simulink model "FULL_IM_HESS"  (R2017b)
settings: Solver=ode4  StartTime=0.0  StopTime=SIMULPARAM.T_end  FixedStep=SIMULPARAM.Ts  RelTol=1e-3  EnableMultiTasking=on
undefined symbols (not defined in the file): BAT, Bat_current_control, BATCURRENTCONTROL, CHAS, Chopper, d_current_control, DC_bus_voltage_control, DCBUSCONTROL, DCCAP, dCURRENTCONTROL, ENV, Flux_control, FLUXCONTROL, FLUXSTRATEGY, IM, L, q_current_control, qCURRENTCONTROL, SC, SC_current_control, SCCURRENTCONTROL, Speed_control, SPEEDCONTROL, STRATEGY, TRANS
libraries: simulink x3
(part 1 of 2)
settings Model: Creator=Huy  LastModifiedBy=baohu
settings DataIOCC: SaveFormat=Array  SignalLoggingSaveFormat=ModelDataLogs  SaveOutput=off  SignalLogging=off  SaveTime=off
settings OptimizationCC: ExpressionDepthLimit=2147483647  LifeSpan=inf
settings DebuggingCC: AlgebraicLoopMsg=none  SaveWithDisabledLinksMsg=none  UnderspecifiedInitializationDetection=Classic  MergeDetectMultiDrivingBlocksExec=none  MaxConsecutiveZCsMsg=none  SolverPrmCheckMsg=warning  FcnCallInpInsideContextMsg=warning  ModelReferenceDataLoggingMessage=none  ModelReferenceExtraNoncontSigs=none  StateNameClashWarn=warning  SFUnexpectedBacktrackingDiag=warning  SFNoUnconditionalDefaultTransitionDiag=warning  SFExecutionAtInitializationDiag=none
settings HardwareCC: ProdBitPerPointer=32  ProdBitPerSizeT=32  ProdBitPerPtrDiffT=32  ProdLargestAtomicFloat=None  ProdIntDivRoundTo=Undefined  ProdEndianess=Unspecified  ProdWordSize=32  ProdHWDeviceType=32-bit Generic
settings ModelReferenceCC: PropagateSignalLabelsOutOfModel=off
settings CodeAppCC: StateflowObjectComments=on
settings GRTTargetCC: TargetLangStandard=C89/C90 (ANSI)  CombineOutputUpdateFcns=off  GRTInterface=on
settings ConfigComp: CovMetricSettings=dw  CovHtmlReporting=on  CovSaveCumulativeToWorkspaceVar=on  CovSaveSingleToWorkspaceVar=on  CovExternalEMLEnable=off

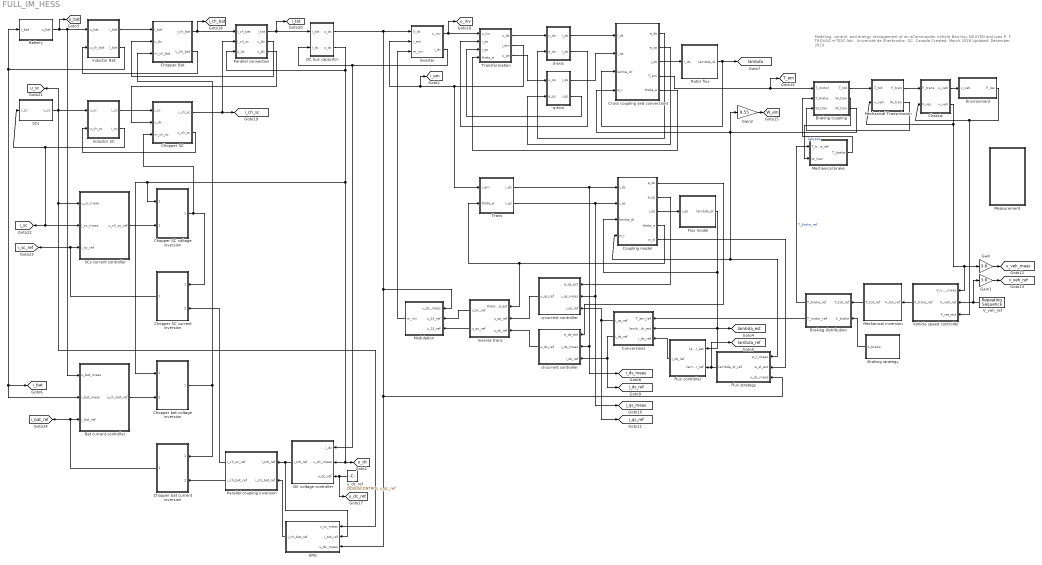
== system FULL_IM_HESS ==
  note: Modeling, control, and energy management of an eCommander vehicle
      | Bao-Huy NGUYEN and Joao P. F. TROVAO
      | e-TESC lab., Université de Sherbrooke, QC, Canada
      | Created: March 2018 Updated: December 2019
  Bat current controller : Subsystem
      mask Display: plot(0,0,100,100, [10,30,90,70,10,90],[90,10,10,90,90,10])
  Battery : Subsystem  AncestorBlock=simulink/REM/SE
      mask Display:
      | plot(0,0,100,100, 1.2*[50,57.68,60.77,63.08,64.97,66.58,68,69.26,70.4, 	71.42,72.36,78.28,80,78.28,72.36,71.42,70.4, 	69.26,68,66.58,64.97,63.08,60.77,57.68,50,42.32, 	39.23,36.92,35.03,33.42,32,30.74,29.6,28.58, 	27.64,21.72,20,21.72,27.64,28.58,29.6,30.74,32, 	33.42,35.03,36.92,39.23,42.32,50]-10, 1.2*[20,21,22,23,24,25,26,27,28,29,30,40,50,60,70,71,72, 	73,74,75,76,77,78,79,80,79,78,77,76,75,74,73,72, 	71,70,60,50,40,30,29,28,27,26,25,24,23,22,21,20]-10)
      | disp('ES')
  Braking coupling : Subsystem  mask(CM){}
      mask Display: plot(0,0,100,100,[35,35,95,95,35],[65,10,10,65,65], [5,5,65,65,5],[90,35,35,90,90])
  Braking distribution : Subsystem  AncestorBlock=simulink/SMC/Bloc de répartition
      mask Display: plot(0,0,100,100,[20,40,100,80,20],[75,20,20,75,75], [0,20,80,60,0],[85,30,30,85,85])
  Braking strategy : Subsystem  AncestorBlock=simulink/SMC/Inversion EC avec mesure
      mask Display: plot(0,0,100,100,[10,30,90,70,10],[90,10,10,90,90])
  Chassis : Subsystem  AncestorBlock=simulink/REM/EA  mask(CM){}
      mask Display: plot(0,0,100,100,[10,10,90,90,10],[90,10,10,90,90], [10,90],[10,90])
  Chopper Bat : Subsystem  AncestorBlock=simulink/REM/EC Elec  mask(Hacheur){}
      mask Display: plot(0,0,100,100,[10,10,90,90,10],[90,10,10,90,90])
  Chopper SC : Subsystem  AncestorBlock=simulink/REM/EC Elec  mask(Hacheur){}
      mask Display: plot(0,0,100,100,[10,10,90,90,10],[90,10,10,90,90])
  Chopper SC current inversion : Subsystem
      mask Display: plot(0,0,100,100,[10,30,90,70,10],[90,10,10,90,90])
  Chopper SC voltage inversion : Subsystem
      mask Display: plot(0,0,100,100,[10,30,90,70,10],[90,10,10,90,90])
  Chopper bat current inversion : Subsystem
      mask Display: plot(0,0,100,100,[10,30,90,70,10],[90,10,10,90,90])
  Chopper bat voltage inversion : Subsystem
      mask Display: plot(0,0,100,100,[10,30,90,70,10],[90,10,10,90,90])
  Conversions : Subsystem  AncestorBlock=simulink/SMC/Bloc de répartition
      mask Display: plot(0,0,100,100,[20,40,100,80,20],[75,20,20,75,75], [0,20,80,60,0],[85,30,30,85,85])
  Coupling model : Subsystem  AncestorBlock=simulink/REM/EC EM
      mask Display: plot(0,0,100,100, [50,57.68,60.77,63.08,64.97,66.58,68,69.26,70.4, 	71.42,72.36,78.28,80,78.28,72.36,71.42,70.4, 	69.26,68,66.58,64.97,63.08,60.77,57.68,50,42.32, 	39.23,36.92,35.03,33.42,32,30.74,29.6,28.58, 	27.64,21.72,20,21.72,27.64,28.58,29.6,30.74,32, 	33.42,35.03,36.92,39.23,42.32,50], [20,21,22,23,24,25,26,27,28,29,30,40,50,60,70,71,72, 	73,74,75,76,77,78,79,80,79,78,77,76,75,74,73,72, 	71,70,60,50,40,30,29,28,27,26,25,24,23,22,21,20]-15,  [50,57.68,60.77,63.08,64.97,66.58,68,69.26,70.4, 	71.42,72.36,78.28,80,78.28,72.36,71.42,70.4, 	69.26,68,66.58,64.97,63.08,60.77,57.68,50,42.32, 	39.23,36.92,35.03,33.42,32,30.74,29.6,28.58, 	27.64,21.72,20,21.72,27.64,28.58,29.6,30.74,32, 	33.42,35.03,36.92,39.23,42.32,50], [20,21,22,23,24,25,26,27,28,29,30,40,50,60,70,71,72, 	73,74,75,76,77,78,79,80,79,78,77,76,75,74,73,72, 	71,70,60,50,40,30,29,28,27,26,25,24,23,22,21,20]+15)
  Cross coupling and conversions : Subsystem  mask(CM){}
      mask Display: plot(0,0,100,100, [50,57.68,60.77,63.08,64.97,66.58,68,69.26,70.4, 	71.42,72.36,78.28,80,78.28,72.36,71.42,70.4, 	69.26,68,66.58,64.97,63.08,60.77,57.68,50,42.32, 	39.23,36.92,35.03,33.42,32,30.74,29.6,28.58, 	27.64,21.72,20,21.72,27.64,28.58,29.6,30.74,32, 	33.42,35.03,36.92,39.23,42.32,50], [20,21,22,23,24,25,26,27,28,29,30,40,50,60,70,71,72, 	73,74,75,76,77,78,79,80,79,78,77,76,75,74,73,72, 	71,70,60,50,40,30,29,28,27,26,25,24,23,22,21,20]-15,  [50,57.68,60.77,63.08,64.97,66.58,68,69.26,70.4, 	71.42,72.36,78.28,80,78.28,72.36,71.42,70.4, 	69.26,68,66.58,64.97,63.08,60.77,57.68,50,42.32, 	39.23,36.92,35.03,33.42,32,30.74,29.6,28.58, 	27.64,21.72,20,21.72,27.64,28.58,29.6,30.74,32, 	33.42,35.03,36.92,39.23,42.32,50], [20,21,22,23,24,25,26,27,28,29,30,40,50,60,70,71,72, 	73,74,75,76,77,78,79,80,79,78,77,76,75,74,73,72, 	71,70,60,50,40,30,29,28,27,26,25,24,23,22,21,20]+15)
  DC bus capacitor : Subsystem  AncestorBlock=simulink/REM/EA  mask(CM){}
      mask Display: plot(0,0,100,100,[10,10,90,90,10],[90,10,10,90,90], [10,90],[10,90])
  DC voltage controller : Subsystem  AncestorBlock=simulink/SMC/Asservissement Correcteur IP
      mask Display: plot(0,0,100,100, [10,30,90,70,10,90],[90,10,10,90,90,10])
  EMS : Subsystem  AncestorBlock=simulink/SMC/Inversion EC avec mesure
      mask Display: plot(0,0,100,100,[10,30,90,70,10],[90,10,10,90,90])
  Environment : Subsystem  AncestorBlock=simulink/REM/SE
      mask Display:
      | plot(0,0,100,100, 1.2*[50,57.68,60.77,63.08,64.97,66.58,68,69.26,70.4, 	71.42,72.36,78.28,80,78.28,72.36,71.42,70.4, 	69.26,68,66.58,64.97,63.08,60.77,57.68,50,42.32, 	39.23,36.92,35.03,33.42,32,30.74,29.6,28.58, 	27.64,21.72,20,21.72,27.64,28.58,29.6,30.74,32, 	33.42,35.03,36.92,39.23,42.32,50]-10, 1.2*[20,21,22,23,24,25,26,27,28,29,30,40,50,60,70,71,72, 	73,74,75,76,77,78,79,80,79,78,77,76,75,74,73,72, 	71,70,60,50,40,30,29,28,27,26,25,24,23,22,21,20]-10)
      | disp('MS')
  Flux controller : Subsystem  AncestorBlock=simulink/SMC/Asservissement Correcteur IP
      mask Display: plot(0,0,100,100, [10,30,90,70,10,90],[90,10,10,90,90,10])
  Flux model : Subsystem  AncestorBlock=simulink/REM/EA  mask(CM){}
      mask Display: plot(0,0,100,100,[10,10,90,90,10],[90,10,10,90,90], [10,90],[10,90])
  Flux strategy : Subsystem  AncestorBlock=simulink/SMC/Inversion EC avec mesure
      mask Display: plot(0,0,100,100,[10,30,90,70,10],[90,10,10,90,90])
  Gain : Gain  Gain=3.6
  Gain1 : Gain  Gain=3.6
  Gain2 : Gain  Gain=9.55
  Inductor Bat : Subsystem  AncestorBlock=simulink/REM/EA  mask(CM){}
      mask Display: plot(0,0,100,100,[10,10,90,90,10],[90,10,10,90,90], [10,90],[10,90])
  Inductor SC : Subsystem  AncestorBlock=simulink/REM/EA  mask(CM){}
      mask Display: plot(0,0,100,100,[10,10,90,90,10],[90,10,10,90,90], [10,90],[10,90])
  Inverse trans : Subsystem  AncestorBlock=simulink/SMC/Bloc de répartition
      mask Display: plot(0,0,100,100,[20,40,100,80,20],[75,20,20,75,75], [0,20,80,60,0],[85,30,30,85,85])
  Inverter : Subsystem  AncestorBlock=simulink/REM/EC Elec  mask(Hacheur){}
      mask Display: plot(0,0,100,100,[10,10,90,90,10],[90,10,10,90,90])
  Measurement : Subsystem
  Mechanical Transmission : Subsystem
      mask Display: plot(0,0,100,100,[10,10,90,90,10],[90,10,10,90,90])
  Mechanical brake : Subsystem  AncestorBlock=simulink/REM/SE
      mask Display:
      | plot(0,0,100,100, 1.2*[50,57.68,60.77,63.08,64.97,66.58,68,69.26,70.4, 	71.42,72.36,78.28,80,78.28,72.36,71.42,70.4, 	69.26,68,66.58,64.97,63.08,60.77,57.68,50,42.32, 	39.23,36.92,35.03,33.42,32,30.74,29.6,28.58, 	27.64,21.72,20,21.72,27.64,28.58,29.6,30.74,32, 	33.42,35.03,36.92,39.23,42.32,50]-10, 1.2*[20,21,22,23,24,25,26,27,28,29,30,40,50,60,70,71,72, 	73,74,75,76,77,78,79,80,79,78,77,76,75,74,73,72, 	71,70,60,50,40,30,29,28,27,26,25,24,23,22,21,20]-10)
      | disp('MS')
  Mechanical inversion : Subsystem  AncestorBlock=simulink/SMC/Inversion EC avec mesure
      mask Display: plot(0,0,100,100,[10,30,90,70,10],[90,10,10,90,90])
  Modulation : Subsystem  AncestorBlock=simulink/SMC/Bloc de répartition
      mask Display: plot(0,0,100,100,[10,30,90,70,10],[90,10,10,90,90])
  Parallel connection : Subsystem  mask(CM){}
      mask Display: plot(0,0,100,100,[35,35,95,95,35],[65,10,10,65,65], [5,5,65,65,5],[90,35,35,90,90])
  Parallel coupling inversion : Subsystem  AncestorBlock=simulink/SMC/Bloc de répartition
      mask Display: plot(0,0,100,100,[20,40,100,80,20],[75,20,20,75,75], [0,20,80,60,0],[85,30,30,85,85])
  Rotor flux : Subsystem  AncestorBlock=simulink/REM/EA  mask(CM){}
      mask Display: plot(0,0,100,100,[10,10,90,90,10],[90,10,10,90,90], [10,90],[10,90])
  SCs : Subsystem  AncestorBlock=simulink/REM/SE
      mask Display:
      | plot(0,0,100,100, 1.2*[50,57.68,60.77,63.08,64.97,66.58,68,69.26,70.4, 	71.42,72.36,78.28,80,78.28,72.36,71.42,70.4, 	69.26,68,66.58,64.97,63.08,60.77,57.68,50,42.32, 	39.23,36.92,35.03,33.42,32,30.74,29.6,28.58, 	27.64,21.72,20,21.72,27.64,28.58,29.6,30.74,32, 	33.42,35.03,36.92,39.23,42.32,50]-10, 1.2*[20,21,22,23,24,25,26,27,28,29,30,40,50,60,70,71,72, 	73,74,75,76,77,78,79,80,79,78,77,76,75,74,73,72, 	71,70,60,50,40,30,29,28,27,26,25,24,23,22,21,20]-10)
      | disp('ES')
  SCs current controller : Subsystem
      mask Display: plot(0,0,100,100, [10,30,90,70,10,90],[90,10,10,90,90,10])
  Trans : Subsystem  mask(CM){}
      mask Display: plot(0,0,100,100,[35,35,95,95,35],[65,10,10,65,65], [5,5,65,65,5],[90,35,35,90,90])
  Transformation : Subsystem  mask(CM){}
      mask Display: plot(0,0,100,100,[35,35,95,95,35],[65,10,10,65,65], [5,5,65,65,5],[90,35,35,90,90])
  V_veh_ref : simulink/Sources/Repeating Sequence  rep_seq_t=CYCL.time  rep_seq_y=CYCL.velocity  mask(Repeating table){}
  Vehicle speed controller : Subsystem  AncestorBlock=simulink/SMC/Asservissement Correcteur IP
      mask Display: plot(0,0,100,100, [10,30,90,70,10,90],[90,10,10,90,90,10])
  d-axis : Subsystem  AncestorBlock=simulink/REM/EA  mask(CM){}
      mask Display: plot(0,0,100,100,[10,10,90,90,10],[90,10,10,90,90], [10,90],[10,90])
  d-current controller : Subsystem  AncestorBlock=simulink/SMC/Asservissement Correcteur IP
      mask Display: plot(0,0,100,100, [10,30,90,70,10,90],[90,10,10,90,90,10])
  q-axis : Subsystem  AncestorBlock=simulink/REM/EA  mask(CM){}
      mask Display: plot(0,0,100,100,[10,10,90,90,10],[90,10,10,90,90], [10,90],[10,90])
  q-current controller : Subsystem  AncestorBlock=simulink/SMC/Asservissement Correcteur IP
      mask Display: plot(0,0,100,100, [10,30,90,70,10,90],[90,10,10,90,90,10])
  u_dc_ref : Constant  Value=DCBUSCONTROL.u_dc_ref
  tag scope: T_em=global, W_em=global, i_bat=global, i_bat_ref=global, i_ch_bat=global, i_ch_sc=global, i_ds_meas=global, i_ds_ref=global, i_em=global, i_qs_meas=global, i_qs_ref=global, i_sc=global, i_sc_ref=global, i_tot=global, lambda=global, lambda_est=global, lambda_ref=global, u_bat=global, u_dc=global, u_dc_ref=global, u_inv=global, u_sc=global, v_veh_meas=global, v_veh_ref=global
  wires:
  Chassis/1(v_veh) -> Environment/1(v_veh)
  Environment/1(F_res) -> Vehicle speed controller/3(F_res_est), Chassis/2(F_res)
  Chassis/2("v_veh ") -> Mechanical Transmission/2(v_veh), Vehicle speed controller/1(V_veh_meas), Gain/1
  Mechanical Transmission/2(W_tran) -> Braking coupling/3("W_tran  ")
  Braking coupling/1(T_tot) -> Mechanical Transmission/1(T_tot)
  Braking coupling/2(W_tran) -> Mechanical brake/2(W_tran)
  Mechanical brake/1(T_brake) -> Braking coupling/2(T_brake)  "T_brake"
  Mechanical inversion/1(T_tot_ref) -> Braking distribution/1(T_tot_ref)
  V_veh_ref/1 -> Vehicle speed controller/2(V_veh_ref), Gain1/1
  Braking distribution/1(T_brake_ref) -> Mechanical brake/1(T_brake_ref)  "T_brake_ref"
  Braking strategy/1(k_brake) -> Braking distribution/2(k_brake)
  d-axis/2("i_ds ") -> Transformation/2(i_ds)
  q-axis/2("i_qs ") -> Transformation/3(i_qs)
  Rotor flux/1(lambda_dr) -> Cross coupling and conversions/3(lamba_dr), [lambda]
  Cross coupling and conversions/1(e_ds) -> d-axis/2(e_ds)
  Cross coupling and conversions/2(e_qs) -> q-axis/2(e_qs)
  Cross coupling and conversions/4(T_em) -> [T_em], Braking coupling/1(T_motor)
  Cross coupling and conversions/5(theta_e) -> Transformation/4(theta_e)
  Braking distribution/2(T_motor_ref) -> Conversions/1(T_em_ref)
  Trans/1(i_ds) -> Coupling model/1(i_ds), [i_ds_meas], d-current controller/2(i_ds_meas)
  Trans/2(i_qs) -> Coupling model/2(i_qs), [i_qs_meas], q-current controller/2(i_qs_meas)
  Flux model/1(lambda_dr) -> Flux controller/1(lambda_dr_est), [lambda_est], Conversions/2(lambda_dr_est), Coupling model/3(lamba_dr)
  Coupling model/3("i_ds ") -> Flux model/1(i_ds)
  Coupling model/4(theta_e) -> Trans/2(theta_e), Inverse trans/1(theta_e_est)
  Braking coupling/3("W_tran ") -> Flux strategy/1(w_r_meas), Coupling model/4(w_r), Gain2/1, Cross coupling and conversions/4(w_r)
  Flux strategy/1(lambda_dr_ref) -> [lambda_ref], Flux controller/2(lambda_dr_ref)
  Inverse trans/2(u_ac_ref) -> Modulation/3(u_13_ref)
  Modulation/1(m_inv) -> Inverter/3(m_inv)
  q-current controller/1(u_qs_ref) -> Inverse trans/2(u_qs_ref)
  d-current controller/1(u_ds_ref) -> Inverse trans/3(u_ds_ref)
  Coupling model/2(e_qs) -> q-current controller/1(e_qs_est)
  Coupling model/1(e_ds) -> d-current controller/1(e_ds_est)
  Flux controller/1(i_ds_ref) -> Conversions/3(i_ds_ref)
  Transformation/1(u_ds) -> d-axis/1(u_ds)
  Transformation/3(u_qs) -> q-axis/1(u_qs)
  Inverse trans/1(u_bc_ref) -> Modulation/2(u_23_ref)
  Inverter/1(u_inv) -> [u_inv], Transformation/1(u_inv)
  Transformation/2(i_em) -> [i_em], Inverter/2(i_em), Trans/1(i_em)
  DC bus capacitor/1(u_dc) -> EMS/3(u_dc_meas), Flux strategy/3(u_dc_meas), Modulation/1(u_dc_meas), Inverter/1(U_dc)
  Parallel coupling inversion/2(i_ch_bat_ref) -> Chopper bat current inversion/2(i_ch_bat_ref)
  Mechanical Transmission/1(F_tran) -> Chassis/1(F_trans)
  Vehicle speed controller/1(F_trans_ref) -> Mechanical inversion/1(F_tot_ref)
  Conversions/1(i_qs_ref) -> [i_qs_ref], q-current controller/3(i_qs_ref)
  Conversions/2("i_ds_ref  ") -> d-current controller/3(i_ds_ref), [i_ds_ref]
  Cross coupling and conversions/3("i_ds ") -> Rotor flux/1(i_ds)
  Coupling model/5(w_sl) -> Flux strategy/2(w_sl_est)
  d-axis/1(i_ds) -> Cross coupling and conversions/1(i_ds)
  q-axis/1(i_qs) -> Cross coupling and conversions/2(i_qs)
  Gain/1 -> [v_veh_meas]
  Gain1/1 -> [v_veh_ref]
  Gain2/1 -> [W_em]
  Inverter/2(i_dc) -> DC voltage controller/1(i_dc), DC bus capacitor/2(i_dc)
  u_dc_ref/1 -> DC voltage controller/3(u_dc_ref), [u_dc_ref]
  Parallel connection/1(i_tot) -> DC bus capacitor/1(i_tot), [i_tot]
  SCs/1(u_sc) -> Inductor SC/1(u_sc), [u_sc], SCs current controller/1(u_sc_meas), EMS/1(u_sc_meas)
  EMS/1(i_ch_bat_ref) -> Parallel coupling inversion/2("i_ch_bat_ref ")
  DC voltage controller/1(i_tot_ref) -> EMS/2(i_tot_ref), Parallel coupling inversion/1(i_tot_ref)
  Inductor SC/1(i_sc) -> Chopper SC/1(i_sc)
  Parallel connection/3("u_dc ") -> Chopper SC/2(u_dc)
  Chopper SC/2(u_ch_sc) -> Inductor SC/2(u_ch_sc)
  Inductor Bat/1(i_bat) -> Chopper Bat/1(i_bat)
  Parallel connection/2(u_dc) -> Chopper Bat/2(u_dc)
  Chopper Bat/2(u_ch_bat) -> Inductor Bat/2(u_ch_bat)
  Inductor SC/2("i_sc ") -> SCs current controller/2(i_sc_meas), [i_sc], SCs/1(i_sc)
  Inductor Bat/2("i_bat ") -> Bat current controller/2(i_bat_meas), [i_bat], Battery/1(i_bat)
  Battery/1(u_bat) -> Bat current controller/1(u_bat_meas), Inductor Bat/1(u_bat), [u_bat]
  SCs current controller/1(u_ch_sc_ref) -> Chopper SC voltage inversion/2(u_ch_sc_ref)
  Parallel coupling inversion/1(i_ch_sc_ref) -> Chopper SC current inversion/2(i_ch_sc_ref)
  Chopper SC voltage inversion/1(m_ch_sc) -> Chopper SC current inversion/1(m_ch_sc), Chopper SC/3(m_ch_sc)
  Chopper SC current inversion/1(i_sc_ref) -> SCs current controller/3(i_sc_ref), [i_sc_ref]
  Chopper bat current inversion/1(i_bat_ref) -> Bat current controller/3(i_bat_ref), [i_bat_ref]
  Bat current controller/1(u_ch_bat_ref) -> Chopper bat voltage inversion/2(u_ch_bat_ref)
  DC bus capacitor/2("u_dc ") -> Parallel connection/3(" u_dc "), Chopper bat voltage inversion/1(u_dc_meas), Chopper SC voltage inversion/1(u_dc_meas), DC voltage controller/2(u_dc_meas), [u_dc]
  Chopper bat voltage inversion/1(m_ch_bat) -> Chopper Bat/3(m_ch_bat), Chopper bat current inversion/1(m_ch_bat)
  Chopper Bat/1(i_ch_bat) -> Parallel connection/1(i_ch_bat), [i_ch_bat]
  Chopper SC/1(i_ch_sc) -> Parallel connection/2(i_ch_sc), [i_ch_sc]

== system FULL_IM_HESS/Bat current controller ==
  u_bat_meas : Inport
  i_bat_meas : Inport  Port=2
  i_bat_ref : Inport  Port=3
  Constant : Constant  Value=Bat_current_control
  IP controller : Subsystem
  Multiport Switch : MultiPortSwitch  Inputs=2
  PI controller : Subsystem
  Sum2 : Sum  Inputs=+-
  u_ch_bat_ref : Outport  InitialOutput=0
  wires:
  Constant/1 -> Multiport Switch/1
  i_bat_ref/1 -> PI controller/2(i_bat_ref), IP controller/2(i_bat_ref)
  Multiport Switch/1 -> Sum2/2
  PI controller/1(u_ind_bat_ref) -> Multiport Switch/2
  Sum2/1 -> u_ch_bat_ref/1
  i_bat_meas/1 -> IP controller/1(i_bat_meas), PI controller/1(i_bat_meas)
  IP controller/1(u_ind_bat_ref) -> Multiport Switch/3
  u_bat_meas/1 -> Sum2/1

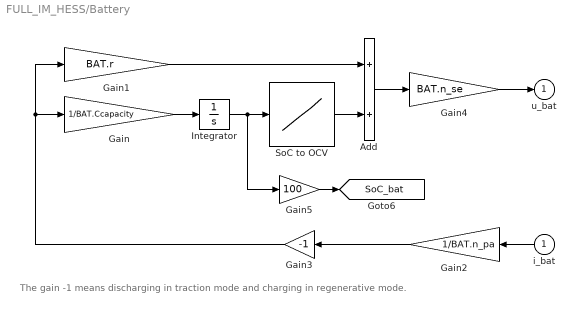
== system FULL_IM_HESS/Battery ==
  note: The gain -1 means discharging in traction mode and charging in regenerative mode.
  i_bat : Inport
  Add : Sum
  Gain : Gain  Gain=1/BAT.Ccapacity
  Gain1 : Gain  Gain=BAT.r
  Gain2 : Gain  Gain=1/BAT.n_pa
  Gain3 : Gain  Gain=-1
  Gain4 : Gain  Gain=BAT.n_se
  Gain5 : Gain  Gain=100
  Integrator : Integrator  InitialCondition=BAT.SoC_init/100
  SoC to OCV : Lookup_n-D  NumberOfTableDimensions=1  BreakpointsForDimension1=0.2:0.1:0.8  Table=11.4:(12-11.4)/((0.8-0.2)/0.1):12  RndMeth=Simplest  InputSameDT=on
  u_bat : Outport  InitialOutput=0
  tag scope: SoC_bat=global
  wires:
  Integrator/1 -> Gain5/1, SoC to OCV/1
  Gain3/1 -> Gain1/1, Gain/1
  Gain/1 -> Integrator/1
  SoC to OCV/1 -> Add/2
  Add/1 -> Gain4/1
  Gain1/1 -> Add/1
  i_bat/1 -> Gain2/1
  Gain4/1 -> u_bat/1
  Gain2/1 -> Gain3/1
  Gain5/1 -> [SoC_bat]

== system FULL_IM_HESS/Braking coupling ==
  T_motor : Inport
  T_brake : Inport  Port=2
  "W_tran  " : Inport  Port=3
  Sum : Sum  Inputs=|+-
  T_tot : Outport  InitialOutput=0
  W_tran : Outport  Port=2  InitialOutput=0
  "W_tran " : Outport  Port=3  InitialOutput=0
  wires:
  T_motor/1 -> Sum/1
  T_brake/1 -> Sum/2
  Sum/1 -> T_tot/1
  "W_tran  "/1 -> W_tran/1, "W_tran "/1

== system FULL_IM_HESS/Braking distribution ==
  T_tot_ref : Inport
  k_brake : Inport  Port=2
  Constant : Constant
  Product : Product  RndMeth=Zero
  Product1 : Product  RndMeth=Zero
  Sum : Sum  Inputs=+-
  T_brake_ref : Outport  InitialOutput=0
  T_motor_ref : Outport  Port=2  InitialOutput=0
  wires:
  Product1/1 -> T_motor_ref/1
  Product/1 -> T_brake_ref/1
  Sum/1 -> Product/2
  T_tot_ref/1 -> Product1/1, Product/1
  k_brake/1 -> Product1/2, Sum/2
  Constant/1 -> Sum/1

== system FULL_IM_HESS/Braking strategy ==
  note: k = 0: Full brake
      | k = 1: Full traction
  Constant : Constant
  k_brake : Outport  InitialOutput=0
  wires:
  Constant/1 -> k_brake/1

== system FULL_IM_HESS/Chassis ==
  F_trans : Inport
  F_res : Inport  Port=2
  Gain : Gain  Gain=1/CHAS.M_veh_tot
  Integrator : Integrator
  Subtract : Sum  Inputs=+-
  v_veh : Outport  InitialOutput=0
  "v_veh " : Outport  Port=2  InitialOutput=0
  wires:
  F_trans/1 -> Subtract/1
  F_res/1 -> Subtract/2
  Subtract/1 -> Gain/1
  Integrator/1 -> v_veh/1, "v_veh "/1
  Gain/1 -> Integrator/1

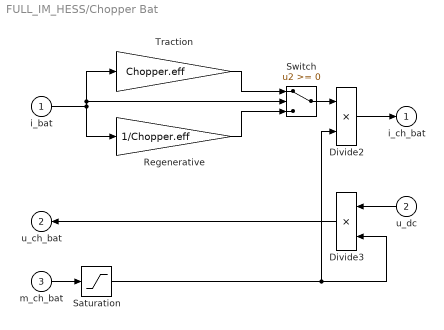
== system FULL_IM_HESS/Chopper Bat ==
  i_bat : Inport
  u_dc : Inport  Port=2
  m_ch_bat : Inport  Port=3
  Divide2 : Product  Inputs=**
  Divide3 : Product  Inputs=**
  Regenerative : Gain  Gain=1/Chopper.eff
  Saturation : Saturate  UpperLimit=1  LowerLimit=0
  Switch : Switch
  Traction : Gain  Gain=Chopper.eff
  i_ch_bat : Outport  InitialOutput=0
  u_ch_bat : Outport  Port=2  InitialOutput=0
  wires:
  m_ch_bat/1 -> Saturation/1
  Regenerative/1 -> Switch/3
  Switch/1 -> Divide2/1
  Saturation/1 -> Divide2/2, Divide3/2
  Traction/1 -> Switch/1
  i_bat/1 -> Traction/1, Switch/2, Regenerative/1
  u_dc/1 -> Divide3/1
  Divide2/1 -> i_ch_bat/1
  Divide3/1 -> u_ch_bat/1

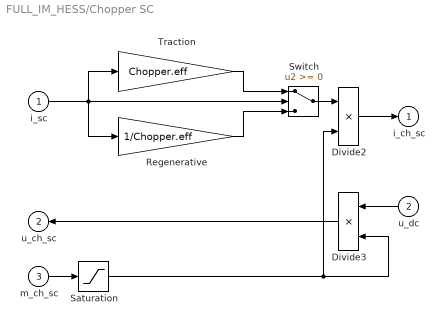
== system FULL_IM_HESS/Chopper SC ==
  i_sc : Inport
  u_dc : Inport  Port=2
  m_ch_sc : Inport  Port=3
  Divide2 : Product  Inputs=**
  Divide3 : Product  Inputs=**
  Regenerative : Gain  Gain=1/Chopper.eff
  Saturation : Saturate  UpperLimit=1  LowerLimit=0
  Switch : Switch
  Traction : Gain  Gain=Chopper.eff
  i_ch_sc : Outport  InitialOutput=0
  u_ch_sc : Outport  Port=2  InitialOutput=0
  wires:
  m_ch_sc/1 -> Saturation/1
  Regenerative/1 -> Switch/3
  Switch/1 -> Divide2/1
  Saturation/1 -> Divide3/2, Divide2/2
  Traction/1 -> Switch/1
  i_sc/1 -> Traction/1, Regenerative/1, Switch/2
  u_dc/1 -> Divide3/1
  Divide2/1 -> i_ch_sc/1
  Divide3/1 -> u_ch_sc/1

== system FULL_IM_HESS/Chopper SC current inversion ==
  m_ch_sc : Inport
  i_ch_sc_ref : Inport  Port=2
  Divide : Product  Inputs=/*
  Memory : Memory  InitialCondition=1
  Regenerative : Gain  Gain=Chopper.eff
  Saturation : Saturate  UpperLimit=1000  LowerLimit=-1000
  Switch : Switch
  Traction : Gain  Gain=1/Chopper.eff
  i_sc_ref : Outport  InitialOutput=0
  wires:
  Divide/1 -> Saturation/1
  Saturation/1 -> i_sc_ref/1
  m_ch_sc/1 -> Memory/1
  Memory/1 -> Divide/1
  Regenerative/1 -> Switch/3
  Traction/1 -> Switch/1
  i_ch_sc_ref/1 -> Regenerative/1, Traction/1, Switch/2
  Switch/1 -> Divide/2

== system FULL_IM_HESS/Chopper SC voltage inversion ==
  u_dc_meas : Inport
  u_ch_sc_ref : Inport  Port=2
  Divide : Product  Inputs=/*
  Saturation : Saturate  UpperLimit=1  LowerLimit=0
  m_ch_sc : Outport  InitialOutput=0
  wires:
  u_ch_sc_ref/1 -> Divide/2
  Divide/1 -> Saturation/1
  Saturation/1 -> m_ch_sc/1
  u_dc_meas/1 -> Divide/1

== system FULL_IM_HESS/Chopper bat current inversion ==
  m_ch_bat : Inport
  i_ch_bat_ref : Inport  Port=2
  Divide : Product  Inputs=/*
  Memory : Memory  InitialCondition=1
  Regenerative : Gain  Gain=Chopper.eff
  Saturation : Saturate  UpperLimit=1000  LowerLimit=-1000
  Switch : Switch
  Traction : Gain  Gain=1/Chopper.eff
  i_bat_ref : Outport  InitialOutput=0
  wires:
  Switch/1 -> Divide/2
  i_ch_bat_ref/1 -> Switch/2, Traction/1, Regenerative/1
  Traction/1 -> Switch/1
  Regenerative/1 -> Switch/3
  Memory/1 -> Divide/1
  m_ch_bat/1 -> Memory/1
  Saturation/1 -> i_bat_ref/1
  Divide/1 -> Saturation/1

== system FULL_IM_HESS/Chopper bat voltage inversion ==
  u_dc_meas : Inport
  u_ch_bat_ref : Inport  Port=2
  Divide : Product  Inputs=/*
  Saturation : Saturate  UpperLimit=1  LowerLimit=0
  m_ch_bat : Outport  InitialOutput=0
  wires:
  u_dc_meas/1 -> Divide/1
  Saturation/1 -> m_ch_bat/1
  Divide/1 -> Saturation/1
  u_ch_bat_ref/1 -> Divide/2

== system FULL_IM_HESS/Conversions ==
  T_em_ref : Inport
  lambda_dr_est : Inport  Port=2
  i_ds_ref : Inport  Port=3
  Constant : Constant  Value=1e-6
  Mux1 : Mux  Inputs=2
  Sum : Sum  Inputs=|++
  i_qs_ref cal : Fcn  Expr=u(1)/((3/2)*IM.pp*(IM.Lm/IM.Lr)*u(2))
  i_qs_ref : Outport  InitialOutput=0
  "i_ds_ref  " : Outport  Port=2  InitialOutput=0
  wires:
  Mux1/1 -> i_qs_ref cal/1
  i_qs_ref cal/1 -> i_qs_ref/1
  i_ds_ref/1 -> "i_ds_ref  "/1
  T_em_ref/1 -> Mux1/1
  lambda_dr_est/1 -> Sum/1
  Sum/1 -> Mux1/2
  Constant/1 -> Sum/2

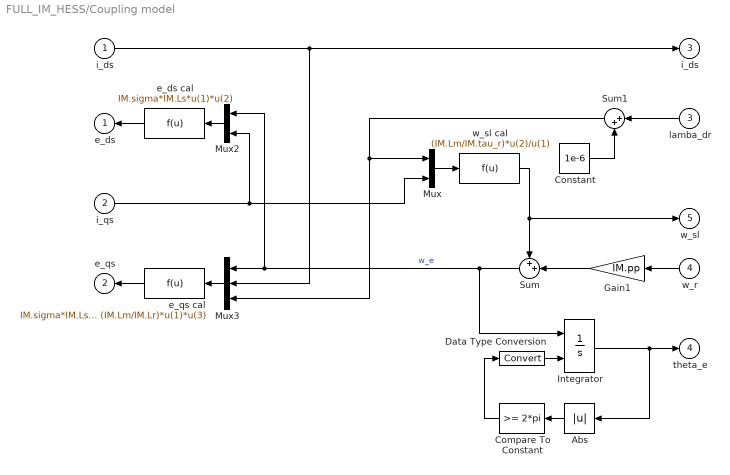
== system FULL_IM_HESS/Coupling model ==
  i_ds : Inport
  i_qs : Inport  Port=2
  lamba_dr : Inport  Port=3
  w_r : Inport  Port=4
  Abs : Abs
  Compare To Constant : simulink/Logic and Bit Operations/Compare To Constant  relop=>=  const=2*pi  OutDataTypeStr=boolean  ZeroCross=off
  Constant : Constant  Value=1e-6
  Data Type Conversion : DataTypeConversion
  Gain1 : Gain  Gain=IM.pp
  Integrator : Integrator  ExternalReset=level
  Mux : Mux  Inputs=2
  Mux2 : Mux  Inputs=2
  Mux3 : Mux  Inputs=3
  Sum : Sum  Inputs=++|
  Sum1 : Sum  Inputs=|++
  e_ds cal : Fcn  Expr=IM.sigma*IM.Ls*u(1)*u(2)
  e_qs cal : Fcn  Expr=IM.sigma*IM.Ls*u(1)*u(2) + (IM.Lm/IM.Lr)*u(1)*u(3)
  w_sl cal : Fcn  Expr=(IM.Lm/IM.tau_r)*u(2)/u(1)
  e_ds : Outport  InitialOutput=0
  e_qs : Outport  Port=2  InitialOutput=0
  "i_ds " : Outport  Port=3  InitialOutput=0
  theta_e : Outport  Port=4  InitialOutput=0
  w_sl : Outport  Port=5  InitialOutput=0
  wires:
  i_ds/1 -> "i_ds "/1, Mux3/2
  Mux/1 -> w_sl cal/1
  i_qs/1 -> Mux2/2, Mux/2
  w_r/1 -> Gain1/1
  w_sl cal/1 -> w_sl/1, Sum/1
  Mux2/1 -> e_ds cal/1
  e_ds cal/1 -> e_ds/1
  Sum/1 -> Integrator/1, Mux2/1, Mux3/1  "w_e"
  Mux3/1 -> e_qs cal/1
  e_qs cal/1 -> e_qs/1
  Sum1/1 -> Mux/1, Mux3/3
  lamba_dr/1 -> Sum1/1
  Constant/1 -> Sum1/2
  Integrator/1 -> theta_e/1, Abs/1
  Abs/1 -> Compare To Constant/1
  Compare To Constant/1 -> Data Type Conversion/1
  Data Type Conversion/1 -> Integrator/2
  Gain1/1 -> Sum/2

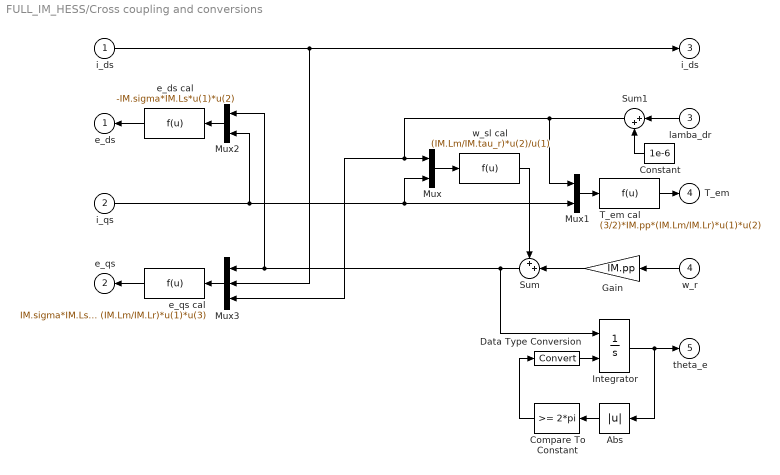
== system FULL_IM_HESS/Cross coupling and conversions ==
  i_ds : Inport
  i_qs : Inport  Port=2
  lamba_dr : Inport  Port=3
  w_r : Inport  Port=4
  Abs : Abs
  Compare To Constant : simulink/Logic and Bit Operations/Compare To Constant  relop=>=  const=2*pi  OutDataTypeStr=boolean  ZeroCross=off
  Constant : Constant  Value=1e-6
  Data Type Conversion : DataTypeConversion
  Gain : Gain  Gain=IM.pp
  Integrator : Integrator  ExternalReset=level
  Mux : Mux  Inputs=2
  Mux1 : Mux  Inputs=2
  Mux2 : Mux  Inputs=2
  Mux3 : Mux  Inputs=3
  Sum : Sum  Inputs=++|
  Sum1 : Sum  Inputs=|++
  T_em cal : Fcn  Expr=(3/2)*IM.pp*(IM.Lm/IM.Lr)*u(1)*u(2)
  e_ds cal : Fcn  Expr=-IM.sigma*IM.Ls*u(1)*u(2)
  e_qs cal : Fcn  Expr=IM.sigma*IM.Ls*u(1)*u(2) + (IM.Lm/IM.Lr)*u(1)*u(3)
  w_sl cal : Fcn  Expr=(IM.Lm/IM.tau_r)*u(2)/u(1)
  e_ds : Outport  InitialOutput=0
  e_qs : Outport  Port=2  InitialOutput=0
  "i_ds " : Outport  Port=3  InitialOutput=0
  T_em : Outport  Port=4  InitialOutput=0
  theta_e : Outport  Port=5  InitialOutput=0
  wires:
  Mux3/1 -> e_qs cal/1
  Integrator/1 -> theta_e/1, Abs/1
  Compare To Constant/1 -> Data Type Conversion/1
  lamba_dr/1 -> Sum1/1
  e_qs cal/1 -> e_qs/1
  Gain/1 -> Sum/2
  Sum1/1 -> Mux1/1, Mux/1, Mux3/3
  i_qs/1 -> Mux/2, Mux1/2, Mux2/2
  Data Type Conversion/1 -> Integrator/2
  Mux2/1 -> e_ds cal/1
  T_em cal/1 -> T_em/1
  Mux1/1 -> T_em cal/1
  e_ds cal/1 -> e_ds/1
  w_r/1 -> Gain/1
  Abs/1 -> Compare To Constant/1
  Constant/1 -> Sum1/2
  Sum/1 -> Mux2/1, Mux3/1, Integrator/1
  i_ds/1 -> "i_ds "/1, Mux3/2
  Mux/1 -> w_sl cal/1
  w_sl cal/1 -> Sum/1

== system FULL_IM_HESS/DC bus capacitor ==
  i_tot : Inport
  i_dc : Inport  Port=2
  Gain : Gain  Gain=1/DCCAP.C
  Integrator : Integrator  InitialCondition=DCCAP.U_init
  Sum : Sum  Inputs=|+-
  u_dc : Outport  InitialOutput=0
  "u_dc " : Outport  Port=2  InitialOutput=0
  wires:
  i_dc/1 -> Sum/2
  Integrator/1 -> "u_dc "/1, u_dc/1
  Sum/1 -> Gain/1
  i_tot/1 -> Sum/1
  Gain/1 -> Integrator/1

== system FULL_IM_HESS/DC voltage controller ==
  i_dc : Inport
  u_dc_meas : Inport  Port=2
  u_dc_ref : Inport  Port=3
  Constant : Constant  Value=DC_bus_voltage_control
  IP controller : Subsystem
  Multiport Switch : MultiPortSwitch  Inputs=2
  PI controller : Subsystem
  Sum : Sum
  i_tot_ref : Outport  InitialOutput=0
  wires:
  PI controller/1(i_c_ref) -> Multiport Switch/2
  Multiport Switch/1 -> Sum/2
  IP controller/1(i_c_ref) -> Multiport Switch/3
  i_dc/1 -> Sum/1
  u_dc_ref/1 -> PI controller/2(u_dc_ref), IP controller/2(u_dc_ref)
  Sum/1 -> i_tot_ref/1
  u_dc_meas/1 -> IP controller/1(u_dc_meas), PI controller/1(u_dc_meas)
  Constant/1 -> Multiport Switch/1

== system FULL_IM_HESS/EMS ==
  u_sc_meas : Inport
  i_tot_ref : Inport  Port=2
  u_dc_meas : Inport  Port=3
  Conventional strategy : Subsystem
  LQR : Subsystem
  Limitation : Subsystem
  i_ch_bat_ref : Outport  InitialOutput=0
  wires:
  u_sc_meas/1 -> LQR/1(u_sc_meas), Limitation/2(u_sc_meas), Conventional strategy/2(u_sc_meas)
  i_tot_ref/1 -> Limitation/1(i_tot_ref), Conventional strategy/1(i_tot_ref)
  LQR/1(i_ch_bat_ref_cal) -> Limitation/3(i_ch_bat_ref_cal)
  Limitation/1(i_ch_bat_ref) -> i_ch_bat_ref/1
  u_dc_meas/1 -> LQR/2(u_dc_meas)

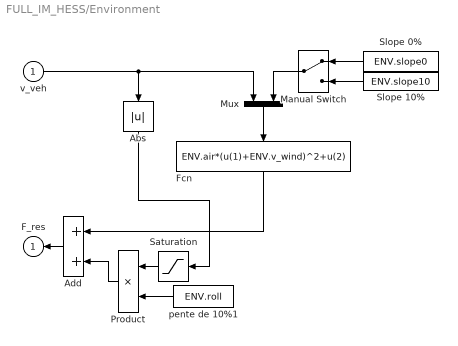
== system FULL_IM_HESS/Environment ==
  v_veh : Inport
  Abs : Abs
  Add : Sum
  Fcn : Fcn  Expr=ENV.air*(u(1)+ENV.v_wind)^2+u(2)
  Manual Switch : ManualSwitch
  Mux : Mux  Inputs=2
  Product : Product  RndMeth=Zero
  Saturation : Saturate  UpperLimit=1  LowerLimit=0
  Slope 0% : Constant  Value=ENV.slope0
  Slope 10% : Constant  Value=ENV.slope10
  pente de 10%1 : Constant  Value=ENV.roll
  F_res : Outport  InitialOutput=0
  wires:
  v_veh/1 -> Mux/1, Abs/1
  Mux/1 -> Fcn/1
  Manual Switch/1 -> Mux/2
  Slope 0%/1 -> Manual Switch/1
  Slope 10%/1 -> Manual Switch/2
  Add/1 -> F_res/1
  Fcn/1 -> Add/1
  pente de 10%1/1 -> Product/2
  Product/1 -> Add/2
  Abs/1 -> Saturation/1
  Saturation/1 -> Product/1

== system FULL_IM_HESS/Flux controller ==
  lambda_dr_est : Inport
  lambda_dr_ref : Inport  Port=2
  Constant : Constant  Value=Flux_control
  IP controller : Subsystem
  Multiport Switch : MultiPortSwitch  Inputs=2
  PI controller : Subsystem
  i_ds_ref : Outport  InitialOutput=0
  wires:
  lambda_dr_est/1 -> IP controller/1(lambda_dr_est), PI controller/1(lambda_dr_est)
  lambda_dr_ref/1 -> IP controller/2(lambda_dr_ref), PI controller/2(lambda_dr_ref)
  Constant/1 -> Multiport Switch/1
  IP controller/1(i_ds_ref) -> Multiport Switch/3
  PI controller/1(i_ds_ref) -> Multiport Switch/2
  Multiport Switch/1 -> i_ds_ref/1

== system FULL_IM_HESS/Flux model ==
  i_ds : Inport
  Magnetization : TransferFcn  Numerator=[IM.Lm]  Denominator=[IM.tau_r 1]
  lambda_dr : Outport  InitialOutput=0
  wires:
  i_ds/1 -> Magnetization/1
  Magnetization/1 -> lambda_dr/1

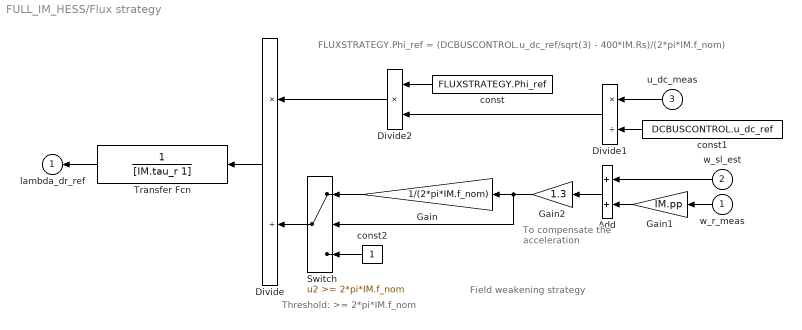
== system FULL_IM_HESS/Flux strategy ==
  note: Field weakening strategy
  note: To compensate
      | the acceleration
  note: FLUXSTRATEGY.Phi_ref = (DCBUSCONTROL.u_dc_ref/sqrt(3) - 400*IM.Rs)/(2*pi*IM.f_nom)
  note: Threshold: >= 2*pi*IM.f_nom
  w_r_meas : Inport
  w_sl_est : Inport  Port=2
  u_dc_meas : Inport  Port=3
  Add : Sum
  Divide : Product  Inputs=*/
  Divide1 : Product  Inputs=*/
  Divide2 : Product  Inputs=**
  Gain : Gain  Gain=1/(2*pi*IM.f_nom)
  Gain1 : Gain  Gain=IM.pp
  Gain2 : Gain  Gain=1.3
  Switch : Switch  Threshold=2*pi*IM.f_nom
  Transfer Fcn : TransferFcn  Denominator=[IM.tau_r 1]
  const : Constant  Value=FLUXSTRATEGY.Phi_ref
  const1 : Constant  Value=DCBUSCONTROL.u_dc_ref
  const2 : Constant
  lambda_dr_ref : Outport  InitialOutput=0
  wires:
  w_r_meas/1 -> Gain1/1
  Add/1 -> Gain2/1
  Gain1/1 -> Add/2
  w_sl_est/1 -> Add/1
  const1/1 -> Divide1/2
  u_dc_meas/1 -> Divide1/1
  Divide1/1 -> Divide2/2
  const/1 -> Divide2/1
  Divide2/1 -> Divide/1
  Gain/1 -> Switch/1
  Switch/1 -> Divide/2
  const2/1 -> Switch/3
  Gain2/1 -> Switch/2, Gain/1
  Divide/1 -> Transfer Fcn/1
  Transfer Fcn/1 -> lambda_dr_ref/1

== system FULL_IM_HESS/Inductor Bat ==
  u_bat : Inport
  u_ch_bat : Inport  Port=2
  Inductor Bat : TransferFcn  Denominator=[L.BAT.L L.BAT.r]
  Sum : Sum  Inputs=|+-
  i_bat : Outport  InitialOutput=0
  "i_bat " : Outport  Port=2  InitialOutput=0
  wires:
  u_ch_bat/1 -> Sum/2
  Inductor Bat/1 -> "i_bat "/1, i_bat/1
  Sum/1 -> Inductor Bat/1
  u_bat/1 -> Sum/1

== system FULL_IM_HESS/Inductor SC ==
  u_sc : Inport
  u_ch_sc : Inport  Port=2
  Inductor SC : TransferFcn  Denominator=[L.SC.L L.SC.r]
  Sum : Sum  Inputs=|+-
  i_sc : Outport  InitialOutput=0
  "i_sc " : Outport  Port=2  InitialOutput=0
  wires:
  u_sc/1 -> Sum/1
  Sum/1 -> Inductor SC/1
  Inductor SC/1 -> i_sc/1, "i_sc "/1
  u_ch_sc/1 -> Sum/2

== system FULL_IM_HESS/Inverse trans ==
  theta_e_est : Inport
  u_qs_ref : Inport  Port=2
  u_ds_ref : Inport  Port=3
  dq2line voltage : Subsystem
  u_bc_ref : Outport  InitialOutput=0
  u_ac_ref : Outport  Port=2  InitialOutput=0
  wires:
  dq2line voltage/2(2) -> u_bc_ref/1
  dq2line voltage/1(1) -> u_ac_ref/1
  theta_e_est/1 -> dq2line voltage/3(theta)
  u_qs_ref/1 -> dq2line voltage/2(q)
  u_ds_ref/1 -> dq2line voltage/1(d)

== system FULL_IM_HESS/Inverter ==
  U_dc : Inport
  i_em : Inport  Port=2
  m_inv : Inport  Port=3
  Divide : Product  Inputs=**
  Divide1 : Product  Inputs=**
  Saturation : Saturate  UpperLimit=1  LowerLimit=-1
  Sum of Elements : Sum  Inputs=+
  u_inv : Outport  InitialOutput=0
  i_dc : Outport  Port=2  InitialOutput=0
  wires:
  i_em/1 -> Divide1/1
  m_inv/1 -> Saturation/1
  Divide/1 -> u_inv/1
  U_dc/1 -> Divide/1
  Sum of Elements/1 -> i_dc/1
  Divide1/1 -> Sum of Elements/1
  Saturation/1 -> Divide/2, Divide1/2

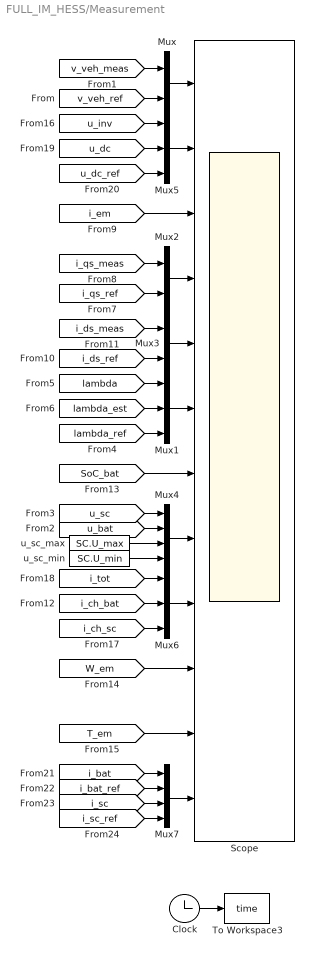
== system FULL_IM_HESS/Measurement ==
  Clock : Clock
      settings: Decimation=10000
  Mux : Mux  Inputs=2
  Mux1 : Mux  Inputs=3
  Mux2 : Mux  Inputs=2
  Mux3 : Mux  Inputs=2
  Mux4 : Mux
  Mux5 : Mux  Inputs=3
  Mux6 : Mux  Inputs=3
  Mux7 : Mux
  Scope : Scope  NumInputPorts=12
  To Workspace3 : ToWorkspace  VariableName=time  SampleTime=-1
      settings: Decimation=SIMULPARAM.Decimation
  u_sc_max : Constant  Value=SC.U_max
  u_sc_min : Constant  Value=SC.U_min
  wires:
  Clock/1 -> To Workspace3/1
  [i_em] -> Scope/3
  [i_ds_meas] -> Mux3/1
  [lambda_ref] -> Mux1/3
  [SoC_bat] -> Scope/7
  [i_qs_meas] -> Mux2/1
  Mux2/1 -> Scope/4
  [i_qs_ref] -> Mux2/2
  [lambda] -> Mux1/1
  [i_ds_ref] -> Mux3/2
  [W_em] -> Scope/10
  [lambda_est] -> Mux1/2
  [v_veh_meas] -> Mux/1
  [v_veh_ref] -> Mux/2
  Mux1/1 -> Scope/6
  Mux/1 -> Scope/1
  [T_em] -> Scope/11
  Mux3/1 -> Scope/5
  [u_dc] -> Mux5/2
  [i_tot] -> Mux6/1
  [u_inv] -> Mux5/1
  u_sc_max/1 -> Mux4/3
  u_sc_min/1 -> Mux4/4
  [u_sc] -> Mux4/1
  [u_bat] -> Mux4/2
  Mux5/1 -> Scope/2
  [i_ch_sc] -> Mux6/3
  Mux4/1 -> Scope/8
  Mux6/1 -> Scope/9
  [u_dc_ref] -> Mux5/3
  [i_ch_bat] -> Mux6/2
  [i_sc] -> Mux7/3
  [i_bat_ref] -> Mux7/2
  [i_sc_ref] -> Mux7/4
  Mux7/1 -> Scope/12
  [i_bat] -> Mux7/1

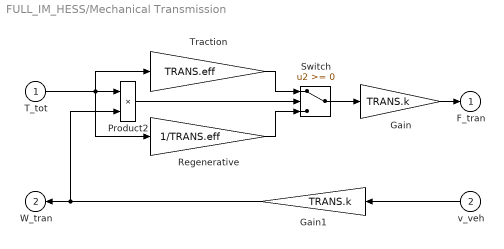
== system FULL_IM_HESS/Mechanical Transmission ==
  T_tot : Inport
  v_veh : Inport  Port=2
  Gain : Gain  Gain=TRANS.k
  Gain1 : Gain  Gain=TRANS.k
  Product2 : Product  RndMeth=Zero
  Regenerative : Gain  Gain=1/TRANS.eff
  Switch : Switch
  Traction : Gain  Gain=TRANS.eff
  F_tran : Outport  InitialOutput=0
  W_tran : Outport  Port=2  InitialOutput=0
  wires:
  T_tot/1 -> Product2/1, Regenerative/1, Traction/1
  Gain/1 -> F_tran/1
  Gain1/1 -> W_tran/1, Product2/2
  v_veh/1 -> Gain1/1
  Product2/1 -> Switch/2
  Traction/1 -> Switch/1
  Regenerative/1 -> Switch/3
  Switch/1 -> Gain/1

== system FULL_IM_HESS/Mechanical brake ==
  T_brake_ref : Inport
  W_tran : Inport  Port=2
  Terminator : Terminator
  T_brake : Outport  InitialOutput=0
  wires:
  T_brake_ref/1 -> T_brake/1
  W_tran/1 -> Terminator/1

== system FULL_IM_HESS/Mechanical inversion ==
  F_tot_ref : Inport
  K_cm : Gain  Gain=1/TRANS.k  SaturateOnIntegerOverflow=on  OutDataTypeStr=Inherit: Same as input  ParamDataTypeStr=Inherit: Same as input
  T_tot_ref : Outport  InitialOutput=0
  wires:
  K_cm/1 -> T_tot_ref/1
  F_tot_ref/1 -> K_cm/1

== system FULL_IM_HESS/Modulation ==
  u_dc_meas : Inport
  u_23_ref : Inport  Port=2
  u_13_ref : Inport  Port=3
  Divide : Product  Inputs=/*
  Mux : Mux  Inputs=2
  Saturation : Saturate  UpperLimit=1  LowerLimit=-1
  m_inv : Outport  InitialOutput=0
  wires:
  u_dc_meas/1 -> Divide/1
  Mux/1 -> Divide/2
  u_23_ref/1 -> Mux/2
  u_13_ref/1 -> Mux/1
  Divide/1 -> Saturation/1
  Saturation/1 -> m_inv/1

== system FULL_IM_HESS/Parallel connection ==
  i_ch_bat : Inport
  i_ch_sc : Inport  Port=2
  " u_dc " : Inport  Port=3
  Sum : Sum  Inputs=|++
  i_tot : Outport  InitialOutput=0
  u_dc : Outport  Port=2  InitialOutput=0
  "u_dc " : Outport  Port=3  InitialOutput=0
  wires:
  " u_dc "/1 -> u_dc/1, "u_dc "/1
  Sum/1 -> i_tot/1
  i_ch_bat/1 -> Sum/1
  i_ch_sc/1 -> Sum/2

== system FULL_IM_HESS/Parallel coupling inversion ==
  i_tot_ref : Inport
  "i_ch_bat_ref " : Inport  Port=2
  Sum : Sum  Inputs=|+-
  i_ch_sc_ref : Outport  InitialOutput=0
  i_ch_bat_ref : Outport  Port=2  InitialOutput=0
  wires:
  "i_ch_bat_ref "/1 -> Sum/2, i_ch_bat_ref/1
  i_tot_ref/1 -> Sum/1
  Sum/1 -> i_ch_sc_ref/1

== system FULL_IM_HESS/Rotor flux ==
  i_ds : Inport
  Magnetization : TransferFcn  Numerator=[IM.Lm]  Denominator=[IM.tau_r 1]
  lambda_dr : Outport  InitialOutput=0
  wires:
  i_ds/1 -> Magnetization/1
  Magnetization/1 -> lambda_dr/1

== system FULL_IM_HESS/SCs ==
  note: The gain -1 means discharging in traction mode and charging in regenerative mode.
  i_sc : Inport
  Add : Sum
  Gain : Gain  Gain=1/SC.C_mod
  Gain1 : Gain  Gain=SC.R_mod
  Gain2 : Gain  Gain=1/SC.n_pa
  Gain3 : Gain  Gain=-1
  Gain4 : Gain  Gain=SC.n_se
  Integrator : Integrator  InitialCondition=SC.U_mod_nom
  u_sc : Outport  InitialOutput=0
  wires:
  Gain2/1 -> Gain3/1
  Gain4/1 -> u_sc/1
  i_sc/1 -> Gain2/1
  Gain1/1 -> Add/1
  Add/1 -> Gain4/1
  Integrator/1 -> Add/2
  Gain/1 -> Integrator/1
  Gain3/1 -> Gain/1, Gain1/1

== system FULL_IM_HESS/SCs current controller ==
  u_sc_meas : Inport
  i_sc_meas : Inport  Port=2
  i_sc_ref : Inport  Port=3
  Constant : Constant  Value=SC_current_control
  IP controller : Subsystem
  Multiport Switch : MultiPortSwitch  Inputs=2
  PI controller : Subsystem
  Sum2 : Sum  Inputs=+-
  u_ch_sc_ref : Outport  InitialOutput=0
  wires:
  u_sc_meas/1 -> Sum2/1
  Sum2/1 -> u_ch_sc_ref/1
  IP controller/1(u_ind_SC_ref) -> Multiport Switch/3
  PI controller/1(u_ind_SC_ref) -> Multiport Switch/2
  Constant/1 -> Multiport Switch/1
  i_sc_ref/1 -> PI controller/2(i_SC_ref), IP controller/2(i_SC_ref)
  i_sc_meas/1 -> IP controller/1(i_SC_meas), PI controller/1(i_SC_meas)
  Multiport Switch/1 -> Sum2/2

== system FULL_IM_HESS/Trans ==
  i_em : Inport
  theta_e : Inport  Port=2
  Demux : Demux  Outputs=2
  current line2dq : Subsystem
  i_ds : Outport  InitialOutput=0
  i_qs : Outport  Port=2  InitialOutput=0
  wires:
  i_em/1 -> Demux/1
  Demux/1 -> current line2dq/1(1)
  Demux/2 -> current line2dq/2(2)
  current line2dq/1(d) -> i_ds/1
  current line2dq/2(q) -> i_qs/1
  theta_e/1 -> current line2dq/3(theta)

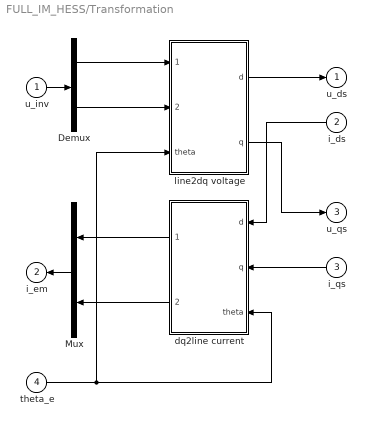
== system FULL_IM_HESS/Transformation ==
  u_inv : Inport
  i_ds : Inport  Port=2
  i_qs : Inport  Port=3
  theta_e : Inport  Port=4
  Demux : Demux  Outputs=2
  Mux : Mux  Inputs=2
  dq2line current : Subsystem
  line2dq voltage : Subsystem
  u_ds : Outport  InitialOutput=0
  i_em : Outport  Port=2  InitialOutput=0
  u_qs : Outport  Port=3  InitialOutput=0
  wires:
  line2dq voltage/1(d) -> u_ds/1
  line2dq voltage/2(q) -> u_qs/1
  i_ds/1 -> dq2line current/1(d)
  i_qs/1 -> dq2line current/2(q)
  u_inv/1 -> Demux/1
  Mux/1 -> i_em/1
  Demux/1 -> line2dq voltage/1(1)
  Demux/2 -> line2dq voltage/2(2)
  theta_e/1 -> line2dq voltage/3(theta), dq2line current/3(theta)
  dq2line current/1(1) -> Mux/1
  dq2line current/2(2) -> Mux/2

== system FULL_IM_HESS/Vehicle speed controller ==
  V_veh_meas : Inport
  V_veh_ref : Inport  Port=2
  F_res_est : Inport  Port=3
  Constant : Constant  Value=Speed_control
  IP controller : Subsystem
  Multiport Switch : MultiPortSwitch  Inputs=2
  PI controller : Subsystem
  Terminator : Terminator
  F_trans_ref : Outport  InitialOutput=0
  wires:
  Multiport Switch/1 -> F_trans_ref/1
  F_res_est/1 -> Terminator/1
  IP controller/1(F_tran_ref) -> Multiport Switch/3
  Constant/1 -> Multiport Switch/1
  V_veh_meas/1 -> IP controller/1(v_veh_meas), PI controller/1(v_veh_meas)
  V_veh_ref/1 -> IP controller/2(v_veh_ref), PI controller/2(v_veh_ref)
  PI controller/1(F_tran_ref) -> Multiport Switch/2

== system FULL_IM_HESS/d-axis ==
  u_ds : Inport
  e_ds : Inport  Port=2
  Sum : Sum  Inputs=|+-
  d-axis : TransferFcn  Denominator=[IM.sigma*IM.Ls IM.Rs]
  i_ds : Outport  InitialOutput=0
  "i_ds " : Outport  Port=2  InitialOutput=0
  wires:
  e_ds/1 -> Sum/2
  d-axis/1 -> "i_ds "/1, i_ds/1
  Sum/1 -> d-axis/1
  u_ds/1 -> Sum/1

== system FULL_IM_HESS/d-current controller ==
  e_ds_est : Inport
  i_ds_meas : Inport  Port=2
  i_ds_ref : Inport  Port=3
  Constant : Constant  Value=d_current_control
  IP controller : Subsystem
  Multiport Switch : MultiPortSwitch  Inputs=2
  PI controller : Subsystem
  Sum2 : Sum  Inputs=++|
  u_ds_ref : Outport  InitialOutput=0
  wires:
  e_ds_est/1 -> Sum2/1
  Sum2/1 -> u_ds_ref/1
  Constant/1 -> Multiport Switch/1
  IP controller/1(u_ds_arm) -> Multiport Switch/3
  PI controller/1(u_ds_arm) -> Multiport Switch/2
  i_ds_meas/1 -> IP controller/1(i_ds_meas), PI controller/1(i_ds_meas)
  i_ds_ref/1 -> IP controller/2(i_ds_ref), PI controller/2(i_ds_ref)
  Multiport Switch/1 -> Sum2/2

== system FULL_IM_HESS/q-axis ==
  u_qs : Inport
  e_qs : Inport  Port=2
  Sum : Sum  Inputs=|+-
  q-axis : TransferFcn  Denominator=[IM.sigma*IM.Ls IM.Rs]
  i_qs : Outport  InitialOutput=0
  "i_qs " : Outport  Port=2  InitialOutput=0
  wires:
  u_qs/1 -> Sum/1
  Sum/1 -> q-axis/1
  q-axis/1 -> i_qs/1, "i_qs "/1
  e_qs/1 -> Sum/2

== system FULL_IM_HESS/q-current controller ==
  e_qs_est : Inport
  i_qs_meas : Inport  Port=2
  i_qs_ref : Inport  Port=3
  Constant : Constant  Value=q_current_control
  IP controller : Subsystem
  Multiport Switch : MultiPortSwitch  Inputs=2
  PI controller : Subsystem
  Sum2 : Sum  Inputs=++|
  u_qs_ref : Outport  InitialOutput=0
  wires:
  e_qs_est/1 -> Sum2/1
  Sum2/1 -> u_qs_ref/1
  Constant/1 -> Multiport Switch/1
  IP controller/1(u_qs_arm) -> Multiport Switch/3
  PI controller/1(u_qs_arm) -> Multiport Switch/2
  i_qs_meas/1 -> IP controller/1(i_qs_meas), PI controller/1(i_qs_meas)
  i_qs_ref/1 -> IP controller/2(i_qs_ref), PI controller/2(i_qs_ref)
  Multiport Switch/1 -> Sum2/2

== system FULL_IM_HESS/Bat current controller/IP controller ==
  i_bat_meas : Inport
  i_bat_ref : Inport  Port=2
  Gain1 : Gain  Gain=BATCURRENTCONTROL.Ki_ip
  Gain2 : Gain  Gain=BATCURRENTCONTROL.Kp_ip
  Integrator : Integrator  IgnoreLimit=on
  Sum : Sum  Inputs=+-
  Sum1 : Sum  Inputs=-+
  u_ind_bat_ref : Outport
  wires:
  Gain2/1 -> Sum/2
  Sum/1 -> u_ind_bat_ref/1
  Integrator/1 -> Sum/1
  i_bat_ref/1 -> Sum1/2
  Gain1/1 -> Integrator/1
  i_bat_meas/1 -> Gain2/1, Sum1/1
  Sum1/1 -> Gain1/1

== system FULL_IM_HESS/Bat current controller/PI controller ==
  i_bat_meas : Inport
  i_bat_ref : Inport  Port=2
  Gain1 : Gain  Gain=BATCURRENTCONTROL.Ki_pi
  Gain2 : Gain  Gain=BATCURRENTCONTROL.Kp_pi
  Integrator : Integrator  IgnoreLimit=on
  Sum : Sum
  Sum1 : Sum  Inputs=-+
  u_ind_bat_ref : Outport
  wires:
  Sum1/1 -> Gain1/1, Gain2/1
  i_bat_meas/1 -> Sum1/1
  Gain1/1 -> Integrator/1
  i_bat_ref/1 -> Sum1/2
  Integrator/1 -> Sum/1
  Sum/1 -> u_ind_bat_ref/1
  Gain2/1 -> Sum/2

== system FULL_IM_HESS/DC voltage controller/IP controller ==
  u_dc_meas : Inport
  u_dc_ref : Inport  Port=2
  Gain : Gain  Gain=DCBUSCONTROL.Kp_ip
  Gain1 : Gain  Gain=DCBUSCONTROL.Ki_ip
  Integrator : Integrator
  Sum1 : Sum  Inputs=-+
  Sum2 : Sum  Inputs=+-
  i_c_ref : Outport
  wires:
  Sum1/1 -> Gain1/1
  u_dc_ref/1 -> Sum1/2
  Gain1/1 -> Integrator/1
  Integrator/1 -> Sum2/1
  Gain/1 -> Sum2/2
  u_dc_meas/1 -> Gain/1, Sum1/1
  Sum2/1 -> i_c_ref/1

== system FULL_IM_HESS/DC voltage controller/PI controller ==
  u_dc_meas : Inport
  u_dc_ref : Inport  Port=2
  Gain : Gain  Gain=DCBUSCONTROL.Kp_pi
  Gain1 : Gain  Gain=DCBUSCONTROL.Ki_pi
  Integrator : Integrator
  Sum1 : Sum  Inputs=-+
  Sum2 : Sum
  i_c_ref : Outport
  wires:
  u_dc_meas/1 -> Sum1/1
  Gain1/1 -> Integrator/1
  Sum1/1 -> Gain1/1, Gain/1
  Gain/1 -> Sum2/2
  Sum2/1 -> i_c_ref/1
  u_dc_ref/1 -> Sum1/2
  Integrator/1 -> Sum2/1

== system FULL_IM_HESS/EMS/Conventional strategy ==
  i_tot_ref : Inport
  u_sc_meas : Inport  Port=2
  1st order filter : TransferFcn  Denominator=[1/(2*pi*STRATEGY.f_c) 1]
  SC recharge : Lookup_n-D  NumberOfTableDimensions=1  BreakpointsForDimension1=[SC.U_min SC.U_max]  Table=[30 10]  InternalRulePriority=Speed  RndMeth=Simplest  InputSameDT=on
  SC recharge logic : Subsystem
  Switch : Switch  Criteria=u2 > Threshold  Threshold=0.5
  i_ch_bat_ref_cal : Outport
  wires:
  SC recharge logic/1(Charge) -> Switch/2
  SC recharge/1 -> Switch/1
  Switch/1 -> 1st order filter/1
  i_tot_ref/1 -> Switch/3, SC recharge logic/1(i_tot_ref)
  u_sc_meas/1 -> SC recharge/1
  1st order filter/1 -> i_ch_bat_ref_cal/1

== system FULL_IM_HESS/EMS/LQR ==
  u_sc_meas : Inport
  u_dc_meas : Inport  Port=2
  Add : Sum  Inputs=+-
  Constant : Constant  Value=SC.U_nom
  Divide : Product  Inputs=**/
  Gain : Gain  Gain=BAT.Q_bat*BAT.n_pa/(SC.U_max-SC.U_min)
  i_ch_bat_ref_cal : Outport
  wires:
  u_sc_meas/1 -> Add/2, Divide/2
  Gain/1 -> Divide/1
  Divide/1 -> i_ch_bat_ref_cal/1
  u_dc_meas/1 -> Divide/3
  Add/1 -> Gain/1
  Constant/1 -> Add/1

== system FULL_IM_HESS/EMS/Limitation ==
  i_tot_ref : Inport
  u_sc_meas : Inport  Port=2
  i_ch_bat_ref_cal : Inport  Port=3
  Add : Sum  Inputs=+-
  Constant3 : Constant
  Divide : Product  Inputs=**
  Divide1 : Product  Inputs=**
  Limitation transition : Subsystem
  Sum : Sum
  i_ch_bat_ref : Outport
  wires:
  i_ch_bat_ref_cal/1 -> Limitation transition/2(i_ch_bat_ref_cal), Divide/1
  i_tot_ref/1 -> Limitation transition/1(i_tot_meas), Divide1/1
  Constant3/1 -> Add/1
  Divide1/1 -> Sum/1
  Divide/1 -> Sum/2
  Add/1 -> Divide/2
  Limitation transition/1(k_d) -> Divide1/2, Add/2
  u_sc_meas/1 -> Limitation transition/3(u_sc_meas)
  Sum/1 -> i_ch_bat_ref/1

== system FULL_IM_HESS/Flux controller/IP controller ==
  lambda_dr_est : Inport
  lambda_dr_ref : Inport  Port=2
  Gain : Gain  Gain=FLUXCONTROL.Kp_ip
  Gain1 : Gain  Gain=FLUXCONTROL.Ki_ip
  Integrator : Integrator
  Sum : Sum  Inputs=+-
  Sum1 : Sum  Inputs=-+
  i_ds_ref : Outport
  wires:
  Sum/1 -> i_ds_ref/1
  Sum1/1 -> Gain1/1
  lambda_dr_est/1 -> Gain/1, Sum1/1
  lambda_dr_ref/1 -> Sum1/2
  Gain1/1 -> Integrator/1
  Integrator/1 -> Sum/1
  Gain/1 -> Sum/2

== system FULL_IM_HESS/Flux controller/PI controller ==
  lambda_dr_est : Inport
  lambda_dr_ref : Inport  Port=2
  Gain : Gain  Gain=FLUXCONTROL.Kp_pi
  Gain1 : Gain  Gain=FLUXCONTROL.Ki_pi
  Integrator : Integrator
  Sum : Sum
  Sum1 : Sum  Inputs=-+
  i_ds_ref : Outport
  wires:
  Gain1/1 -> Integrator/1
  lambda_dr_est/1 -> Sum1/1
  Gain/1 -> Sum/1
  Sum1/1 -> Gain1/1, Gain/1
  Integrator/1 -> Sum/2
  Sum/1 -> i_ds_ref/1
  lambda_dr_ref/1 -> Sum1/2

== system FULL_IM_HESS/Inverse trans/dq2line voltage ==
  d : Inport
  q : Inport  Port=2
  theta : Inport  Port=3
  Add2 : Sum  Inputs=+-
  Add3 : Sum  Inputs=+-
  albe2abc : Subsystem
  dq2albe : Subsystem
  1 : Outport
  2 : Outport  Port=2
  wires:
  dq2albe/1(alpha) -> albe2abc/1(alpha)
  dq2albe/2(beta) -> albe2abc/2(beta)
  albe2abc/2(b) -> Add3/1
  albe2abc/1(a) -> Add2/1
  albe2abc/3(c) -> Add3/2, Add2/2
  Add2/1 -> 1/1
  Add3/1 -> 2/1
  d/1 -> dq2albe/1(d)
  q/1 -> dq2albe/2(q)
  theta/1 -> dq2albe/3(theta)

== system FULL_IM_HESS/SCs current controller/IP controller ==
  i_SC_meas : Inport
  i_SC_ref : Inport  Port=2
  Gain1 : Gain  Gain=SCCURRENTCONTROL.Ki_ip
  Gain2 : Gain  Gain=SCCURRENTCONTROL.Kp_ip
  Integrator : Integrator  IgnoreLimit=on
  Sum : Sum  Inputs=+-
  Sum1 : Sum  Inputs=-+
  u_ind_SC_ref : Outport
  wires:
  Gain2/1 -> Sum/2
  Sum/1 -> u_ind_SC_ref/1
  Integrator/1 -> Sum/1
  i_SC_ref/1 -> Sum1/2
  Gain1/1 -> Integrator/1
  i_SC_meas/1 -> Gain2/1, Sum1/1
  Sum1/1 -> Gain1/1

== system FULL_IM_HESS/SCs current controller/PI controller ==
  i_SC_meas : Inport
  i_SC_ref : Inport  Port=2
  Gain1 : Gain  Gain=SCCURRENTCONTROL.Ki_pi
  Gain2 : Gain  Gain=SCCURRENTCONTROL.Kp_pi
  Integrator : Integrator  IgnoreLimit=on
  Sum : Sum
  Sum1 : Sum  Inputs=-+
  u_ind_SC_ref : Outport
  wires:
  Sum1/1 -> Gain1/1, Gain2/1
  i_SC_meas/1 -> Sum1/1
  Gain1/1 -> Integrator/1
  i_SC_ref/1 -> Sum1/2
  Integrator/1 -> Sum/1
  Sum/1 -> u_ind_SC_ref/1
  Gain2/1 -> Sum/2

== system FULL_IM_HESS/Trans/current line2dq ==
  1 : Inport
  2 : Inport  Port=2
  theta : Inport  Port=3
  Add : Sum  Inputs=--
  abc2albe : Subsystem
  albe2dq : Subsystem
  d : Outport
  q : Outport  Port=2
  wires:
  albe2dq/1(d) -> d/1
  albe2dq/2(q) -> q/1
  abc2albe/1(alpha) -> albe2dq/1(alpha)
  abc2albe/2(beta) -> albe2dq/2(beta)
  theta/1 -> albe2dq/3(theta)
  Add/1 -> abc2albe/3(c)
  2/1 -> abc2albe/2(b), Add/2
  1/1 -> abc2albe/1(a), Add/1

== system FULL_IM_HESS/Transformation/dq2line current ==
  d : Inport
  q : Inport  Port=2
  theta : Inport  Port=3
  Terminator : Terminator
  albe2abc : Subsystem
  dq2albe : Subsystem
  1 : Outport
  2 : Outport  Port=2
  wires:
  dq2albe/1(alpha) -> albe2abc/1(alpha)
  dq2albe/2(beta) -> albe2abc/2(beta)
  albe2abc/1(a) -> 1/1
  albe2abc/2(b) -> 2/1
  d/1 -> dq2albe/1(d)
  q/1 -> dq2albe/2(q)
  theta/1 -> dq2albe/3(theta)
  albe2abc/3(c) -> Terminator/1
